simulink model "convertidor_inversor"  (R2022b)
settings: Solver=VariableStepAuto  StartTime=0.0  StopTime=1  RelTol=1e-3
InitFcn:
  | Ts = 100e-6;
StartFcn:
  | Ts = 100e-6;
undefined symbols (not defined in the file): Ion, Lithium
libraries: spsIGBTDiodeLib x8, slpidlib x7, spsCurrentMeasurementLib x5, spsVoltageMeasurementLib x5, spsThreePhaseSeriesRLCBranchLib x5, spsSeriesRLCBranchLib x4, spsAlphaBetaZerotodq0Lib x3, simulink x3, spsabctoAlphaBetaZeroLib x3, spsDCVoltageSourceLib x2, spsThreePhaseVIMeasurementLib x2, spsBatteryLib x1
(part 2 of 2)

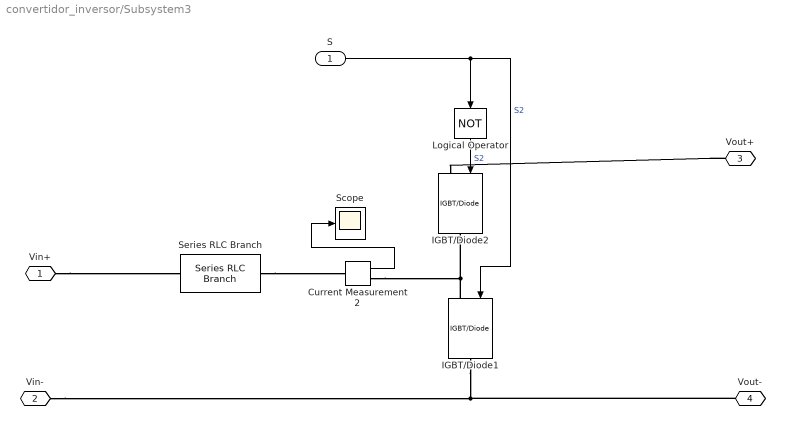
== system convertidor_inversor/Subsystem3 ==
  S : Inport
  Current Measurement2 : spsCurrentMeasurementLib/Current Measurement  PhasorSimulation=off  OutputType=Complex  PSBequivalent=0
  IGBT/Diode1 : spsIGBTDiodeLib/IGBT//Diode  Ron=1e-3  Rs=1e5  Cs=inf  Measurements=off
  IGBT/Diode2 : spsIGBTDiodeLib/IGBT//Diode  Ron=1e-3  Rs=1e5  Cs=inf  Measurements=off
  Logical Operator : Logic  Operator=NOT  AllPortsSameDT=off  OutDataTypeStr=boolean
  Scope : Scope
  Series RLC Branch : spsSeriesRLCBranchLib/Series RLC Branch  LConnTagsString=__new0  RConnTagsString=__new0  BranchType=L  Resistance=3  Inductance=30e-3  SetiL0=off  InitialCurrent=0  Capacitance=1e-6  Setx0=off  InitialVoltage=0  Measurements=None
  Vin+ : PMIOPort  Side=Left
  Vin- : PMIOPort  Port=2  Side=Left
  Vout+ : PMIOPort  Port=3  Side=Right
  Vout- : PMIOPort  Port=4  Side=Right
  wires:
  S/1 -> IGBT/Diode1/1, Logical Operator/1  "S2"
  Logical Operator/1 -> IGBT/Diode2/1  "S2"
  Current Measurement2/1 -> Scope/1
  connections:
  Vin-/RConn1 -- Vout-/RConn1 -- IGBT/Diode1/RConn1
  Series RLC Branch/RConn1 -- Current Measurement2/LConn1
  Vin+/RConn1 -- Series RLC Branch/LConn1
  IGBT/Diode1/LConn1 -- Current Measurement2/RConn1 -- IGBT/Diode2/RConn1
  Vout+/RConn1 -- IGBT/Diode2/LConn1

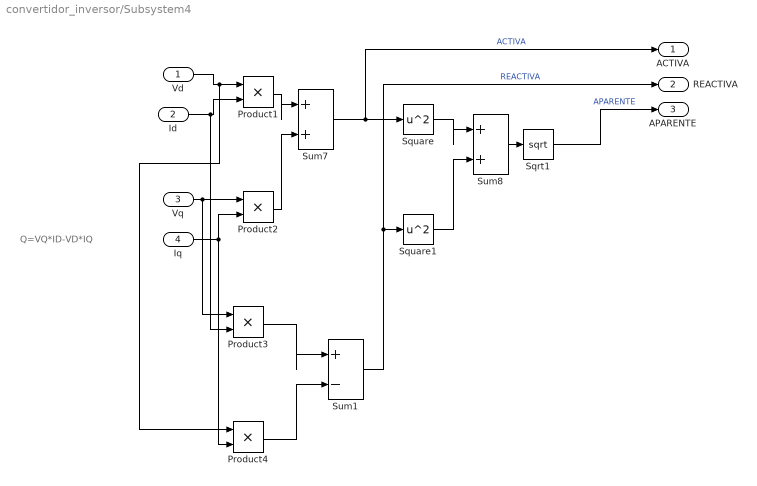
== system convertidor_inversor/Subsystem4 ==
  note: Q=VQ*ID-VD*IQ
  Vd : Inport
  Id : Inport  Port=2
  Vq : Inport  Port=3
  Iq : Inport  Port=4
  Product{1..4} (4 alike) : Product
  Sqrt1 : Sqrt
  Square : Math  Operator=square
  Square1 : Math  Operator=square
  Sum1 : Sum  Inputs=|+-
  Sum7 : Sum  Inputs=|++
  Sum8 : Sum  Inputs=|++
  ACTIVA : Outport
  REACTIVA : Outport  Port=2
  APARENTE : Outport  Port=3
  wires:
  Product1/1 -> Sum7/1
  Product2/1 -> Sum7/2
  Square/1 -> Sum8/1
  Sum7/1 -> ACTIVA/1, Square/1  "ACTIVA"
  Sum8/1 -> Sqrt1/1
  Iq/1 -> Product4/2, Product2/2
  Vq/1 -> Product3/1, Product2/1
  Vd/1 -> Product4/1, Product1/1
  Sqrt1/1 -> APARENTE/1  "APARENTE"
  Id/1 -> Product3/2, Product1/2
  Product3/1 -> Sum1/1
  Product4/1 -> Sum1/2
  Sum1/1 -> REACTIVA/1, Square1/1  "REACTIVA"
  Square1/1 -> Sum8/2

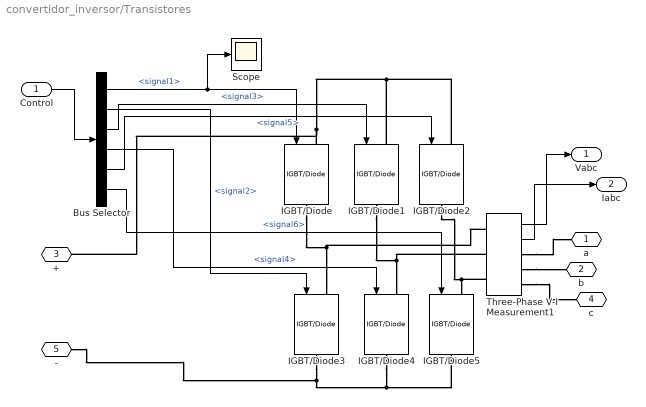
== system convertidor_inversor/Transistores ==
  Control : Inport
  Bus Selector : BusSelector  OutputSignals=signal1,signal2,signal3,signal4,signal5,signal6
  IGBT/Diode{,1..5} (6 alike) : spsIGBTDiodeLib/IGBT//Diode  Ron=1e-3  Rs=1e5  Cs=inf  Measurements=off
  Scope : Scope
  Three-Phase V-I Measurement1 : spsThreePhaseVIMeasurementLib/Three-Phase V-I Measurement  VoltageMeasurement=phase-to-phase  SetLabelV=off  LabelV=Vabc  Vpu=off  VpuLL=off  CurrentMeasurement=yes  SetLabelI=off  LabelI=Iabc  Ipu=off  Pbase=100e6  Vbase=500e3  OutputType=Complex  PhasorSimulation=off  PSBequivalent=0
  a : PMIOPort  Side=Right
  b : PMIOPort  Port=2  Side=Right
  + : PMIOPort  Port=3  Side=Left
  c : PMIOPort  Port=4  Side=Right
  - : PMIOPort  Port=5  Side=Left
  Vabc : Outport
  Iabc : Outport  Port=2
  wires:
  Three-Phase V-I Measurement1/2 -> Iabc/1
  Three-Phase V-I Measurement1/1 -> Vabc/1
  Bus Selector/1 -> IGBT/Diode/1, Scope/1  "<signal1>"
  Control/1 -> Bus Selector/1
  Bus Selector/2 -> IGBT/Diode3/1  "<signal2>"
  Bus Selector/3 -> IGBT/Diode1/1  "<signal3>"
  Bus Selector/4 -> IGBT/Diode4/1  "<signal4>"
  Bus Selector/5 -> IGBT/Diode2/1  "<signal5>"
  Bus Selector/6 -> IGBT/Diode5/1  "<signal6>"
  connections:
  IGBT/Diode/RConn1 -- Three-Phase V-I Measurement1/LConn1 -- IGBT/Diode3/LConn1
  IGBT/Diode1/RConn1 -- Three-Phase V-I Measurement1/LConn2 -- IGBT/Diode4/LConn1
  IGBT/Diode2/RConn1 -- Three-Phase V-I Measurement1/LConn3 -- IGBT/Diode5/LConn1
  IGBT/Diode1/LConn1 -- IGBT/Diode2/LConn1 -- IGBT/Diode/LConn1 -- +/RConn1
  IGBT/Diode3/RConn1 -- -/RConn1 -- IGBT/Diode4/RConn1 -- IGBT/Diode5/RConn1
  Three-Phase V-I Measurement1/RConn3 -- c/RConn1
  Three-Phase V-I Measurement1/RConn1 -- a/RConn1
  Three-Phase V-I Measurement1/RConn2 -- b/RConn1

== matlab function convertidor_inversor/MATLAB Function ==
  data: IN input; COR output; SAL output
%BLOQUE YA HECHO CON EL REPARTO 28/09/2023

function [COR,SAL]    = P_REG(IN)

 persistent val;
 
 if isempty(val)
     val=0;
 end
  
if IN >= 980
    COR =80;
    SAL= true;
    val=1;
elseif IN < 980 && val==1;
    COR =80;
    SAL= true;
else
   COR=0;
   SAL=false;
end
    
 
% 
% function [COR,SAL]    = P_REG(IN)
% 
% persistent dato;
% 
% if isempty(dato)
%     dato=0;
%     
% end
%         
% if IN >= 550
%    dato=dato+10;
%    if dato>=50
%      COR = 80;
%      SAL=true;
%    else
%       COR=0;
%       SAL=false;
%    end      
% else
%    COR=0;
%    SAL=false;
% end
%
